simulink model "DC_control"  (R2024a)
settings: Solver=ode45  StartTime=0.0  StopTime=0.4  RelTol=1e-4
values from neighbouring files (symbols this model uses):
  Va_rated = 140    [set_DC_motor_param.m]
undefined symbols (not defined in the file or in its folder): Kac, Kic, Kpc
settings Model: Creator=CDSL-2  LastModifiedBy=vv

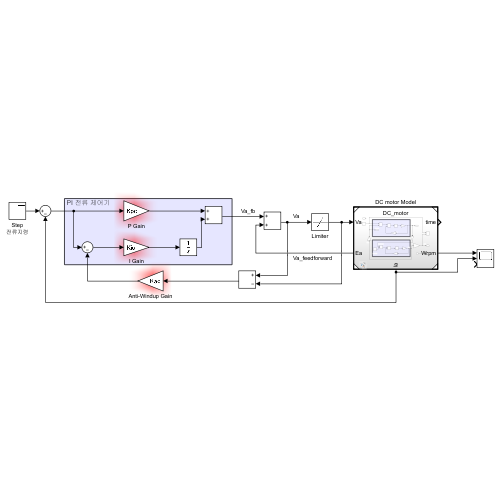
[thumbnail: Simulink's stored preview of the top-level diagram]
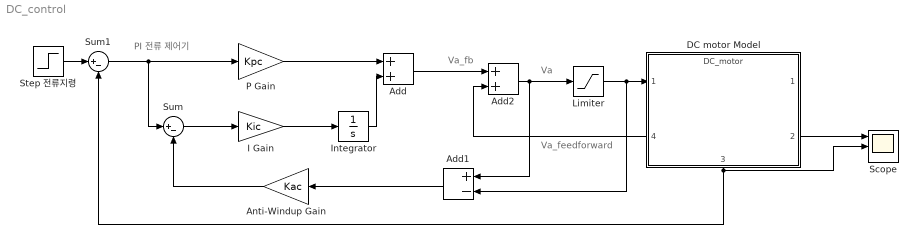
== system DC_control ==
  note: Va_feedforward
  note: Va
  note: Va_fb
  note: PI 전류 제어기
  Add : Sum
  Add1 : Sum  Inputs=+-
  Add2 : Sum
  Anti-Windup Gain : Gain  Gain=Kac
  DC motor Model : ModelReference  ModelNameDialog=DC_motor.slx  SimulationMode=Normal  ModelReferenceVersion=1.32
      settings: PortSchema="{\"entries\":[{\"content\":{\"sides\":[{\"content\":{\"connectorIds\":[\"In1\",\"Out4\"]},\"type\":\"ConnectorPlacement.EquallySpacedRectSide\",\"uuid\":\"2ad6bd00-0316-406a-ba45-d5f6de416ff9\"},{\"content\":{\"connectorIds\":[\"Out1\",\"Out2\"],\"side\":\"RIGHT\"},\"type\":\"ConnectorPlacement.EquallySpacedRectSide\",\"uuid\":\"2fc829f6-4485-4c6c-8a5a-695cf05eae2e\"},{\"content\":{\"side\":\"TOP\"},\"type\":\"ConnectorPlacement.EquallySpacedRectSide\",\"uuid\":\"69e7e481-9ef7-4043-b8a6-02d74540c0e1\"},{\"content\":{\"connectorIds\":[\"Out3\"],\"side\":\"BOTTOM\"},\"type\":\"ConnectorPlacement.EquallySpacedRectSide\",\"uuid\":\"e85b2455-2635-4826-aad7-bdd1458b014d\"}]},\"type\":\"ConnectorPlacement.EquallySpacedConnector\",\"uuid\":\"cdeda118-68f9-4b49-9807-dc0072112b87\"}],\"packageUris\":[\"http://schema.mathworks.com/mf0/Connector/R2020b\"],\"version\":\"1.0\"}"
  I Gain : Gain  Gain=Kic
  Integrator : Integrator
  Limiter : Saturate  UpperLimit=Va_rated  LowerLimit=-Va_rated
  P Gain : Gain  Gain=Kpc
  Scope : Scope  NumInputPorts=3
  Step 전류지령 : Step  Time=0.005  After=20  SampleTime=0
  Sum : Sum  Inputs=|+-
  Sum1 : Sum  Inputs=|+-
  wires:
  I Gain/1 -> Integrator/1
  Integrator/1 -> Add/2
  P Gain/1 -> Add/1
  Sum/1 -> I Gain/1
  Sum1/1 -> Sum/1, P Gain/1
  Add1/1 -> Anti-Windup Gain/1
  Add/1 -> Add2/1
  Add2/1 -> Limiter/1, Add1/1
  Limiter/1 -> Add1/2, DC motor Model/1
  DC motor Model/4 -> Add2/2
  Anti-Windup Gain/1 -> Sum/2
  DC motor Model/3 -> Scope/2, Sum1/2
  Step 전류지령/1 -> Sum1/1
  DC motor Model/2 -> Scope/1
